simulink model "RM3_DD_PTO"  (R2019b)
settings: Solver=ode4  StartTime=0  StopTime=400  FixedStep=0.001  MaxStep=0.001  RelTol=1e-3  EnableMultiTasking=on
values from neighbouring files (symbols this model uses):
  ptosim = ptoSimClass('Direct Drive Linear Generator')    [ptoSimInputFile.m]
undefined symbols (not defined in the file or in its folder): body, constraint, pto
libraries: WECSim_Lib x5
settings Model: Creator=mlawson  LastModifiedBy=ahm_e
settings SolverCC: ZeroCrossControl=DisableAll  AlgebraicLoopSolver=LineSearch  AutoInsertRateTranBlk=on
settings DataIOCC: SaveFormat=Array  SaveOutput=off  SaveTime=off  ReturnWorkspaceOutputs=off
settings OptimizationCC: LifeSpan=inf
settings DebuggingCC: UnderspecifiedInitializationDetection=Classic  MergeDetectMultiDrivingBlocksExec=none  SolverPrmCheckMsg=warning  AllowSymbolicDim=off  StateNameClashWarn=warning  SFUnexpectedBacktrackingDiag=warning  SFNoUnconditionalDefaultTransitionDiag=warning  ArithmeticOperatorsInVariantConditions=warning
settings HardwareCC: ProdBitPerPointer=32  ProdBitPerSizeT=32  ProdBitPerPtrDiffT=32  ProdLargestAtomicFloat=None  ProdIntDivRoundTo=Undefined  ProdEndianess=Unspecified  ProdWordSize=32  ProdHWDeviceType=32-bit Generic
settings ModelReferenceCC: PropagateSignalLabelsOutOfModel=off
settings SFSimCC: SimUseLocalCustomCode=off  CustomCodeUndefinedFunction=UseInterfaceOnly
settings RTWCC: RTWUseLocalCustomCode=off
settings CodeAppCC: StateflowObjectComments=on
settings GRTTargetCC: TargetLangStandard=C89/C90 (ANSI)
settings ConfigComp: CovMetricSettings=dw  CovSaveCumulativeToWorkspaceVar=on  CovSaveSingleToWorkspaceVar=on  CovExternalEMLEnable=off  CovSFcnEnable=off
settings SimscapeCC: SimscapeNormalizeSystem=off
settings ConfigurationSet: Description=SimMechanics 2G
settings ExplorerConfigSet: InternalSimMechanicsExplorerSettings="<ExplorerConfiguration><canonicalview>default</canonicalview><TilePanel><TileInfo><Tiles Columns=\"1\" Count=\"1\" Rows=\"1\"><Column Left=\"2\" Weight=\"1\"/><Column Left=\"1335\"/><Row Top=\"2\" Weight=\"1\"/><Row Top=\"911\"/><Tile Height=\"1\" Width=\"1\" X=\"0\" Y=\"0\"/></Tiles></TileInfo><SceneInfo><SceneViewer><BGColor><R>0.60000002384185791</R><G>0.60000002384185791</G><B>0.60000002384185791</B></BGColor><Camera><Position><X>365.37645888990272</X><Y>-369.82486814446582</Y><Z>359.64809521743916</Z></Position><Center><X>-6.7351450971904585</X><Y>2.2867358426280204</Y><Z>-12.463508769654169</Z></Center><Up><X>-0.40824829046386307</X><Y>0.40824829046386307</Y><Z>0.81649658092772615</Z></Up><Left>-57.820127362122818</Left><Right>57.820127362122818</Right><Bottom>-38.308817187253304</Bottom><Top>38.308817187253304</Top></Camera></SceneViewer></SceneInfo></TilePanel></ExplorerConfiguration>"

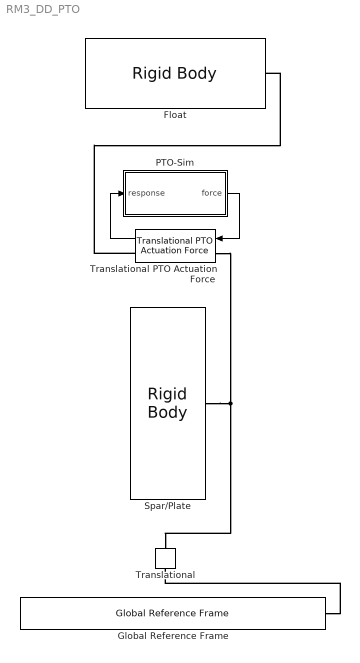
== system RM3_DD_PTO ==
  Float : WECSim_Lib/Body Elements/Rigid Body  body=body(1)
      settings: AttributesFormatString=%<body>  SourceProductName=WEC-Sim
  Global Reference Frame : WECSim_Lib/Frames/Global Reference Frame  waves=waves  simu=simu
      settings: SourceProductName=WEC-Sim
  PTO-Sim : Subsystem
  Spar/Plate : WECSim_Lib/Body Elements/Rigid Body  body=body(2)
      settings: AttributesFormatString=%<body>  SourceProductName=WEC-Sim
  Translational : WECSim_Lib/Constraints/Translational  constraint=constraint(1)
      settings: AttributesFormatString=%<constraint>  SourceProductName=WEC-Sim
  Translational PTO Actuation Force : WECSim_Lib/PTOs/Translational PTO Actuation Force  pto=pto(1)
      settings: AttributesFormatString=%<pto>  SourceProductName=WEC-Sim
  wires:
  Translational PTO Actuation Force/1 -> PTO-Sim/1(response)
  PTO-Sim/1(force) -> Translational PTO Actuation Force/1
  connections:
  Global Reference Frame/RConn1 -- Translational/LConn1
  Spar/Plate/RConn1 -- Translational PTO Actuation Force/LConn1 -- Translational/RConn1
  Translational PTO Actuation Force/RConn1 -- Float/RConn1

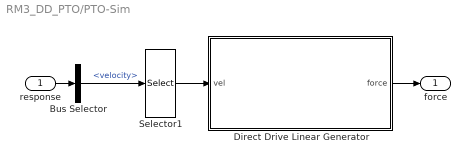
== system RM3_DD_PTO/PTO-Sim ==
  response : Inport
  Bus Selector : BusSelector  OutputSignals=velocity
  Direct Drive Linear Generator : Subsystem  AncestorBlock=PTOSim_Lib/Generator/Direct Drive Linear Generator  mask{ptosim=ptosim.pmLinearGenerator(1)}
      mask prompts: ptosim "Machine Name:"
      mask init:
      | if exist ('ptosim','var')
      |     h = [gcb '/To Workspace'];
      |     responseName = ['pmLinearGenerator' num2str(ptosim.number) '_out'];
      |     set_param(h,'VariableName',responseName);
      |     if ischar(ptosim.Rs)==1 ...
      |        || ischar(ptosim.Bfric)==1 ...
      |        || ischar(ptosim.tau_p)==1 ...
      |        || ischar(ptosim.lambda_fd)==1 ...
      |        || ischar(ptosim.Ls)==1 ...
      |        || ischar(ptosim.theta_d_0)==1 ...
      |        || ischar(ptosim.lambda_sq_0)==1 ...
      |        || ischar(ptosim.lambda_sd_0)==1 ...
      |        || ischar(ptosim.Rload) ==1
      |           error('One of the linear generator variables is undefined. For example, ptosim.pmLinearGenerator.variableName')
      |     end       
      | end
      | clear h responseName
  Selector1 : Selector  InputPortWidth=6  IndexOptions=Index vector (dialog)  Indices=3  OutputSizes=1
  force : Outport  VectorParamsAs1DForOutWhenUnconnected=off
  wires:
  Direct Drive Linear Generator/1(force) -> force/1
  response/1 -> Bus Selector/1
  Bus Selector/1 -> Selector1/1  "<velocity>"
  Selector1/1 -> Direct Drive Linear Generator/1(vel)

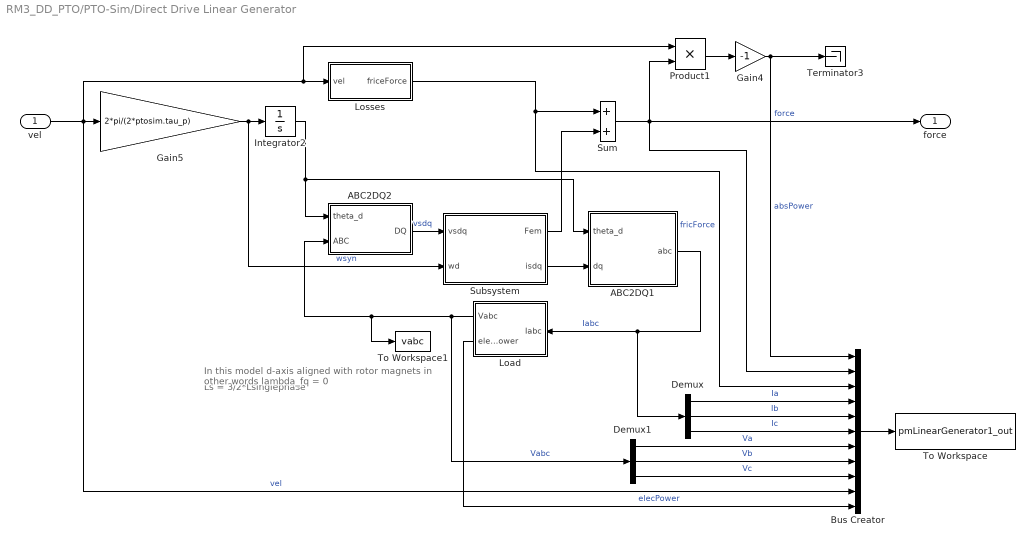
== system RM3_DD_PTO/PTO-Sim/Direct Drive Linear Generator ==
  note: Ls = 3/2*Lsinglephase
  note: In this model d-axis aligned with rotor magnets
      | in other words lambda_fq = 0
  vel : Inport
  ABC2DQ1 : Subsystem
  ABC2DQ2 : Subsystem
  Bus Creator : BusCreator  Inputs=11
  Demux : Demux  Outputs=3
  Demux1 : Demux  Outputs=3
  Gain4 : Gain  Gain=-1
  Gain5 : Gain  Gain=2*pi/(2*ptosim.tau_p)
  Integrator2 : Integrator  InitialCondition=ptosim.theta_d_0
  Load : Subsystem
  Losses : Subsystem
  Product1 : Product
  Subsystem : Subsystem
  Sum : Sum
  Terminator3 : Terminator
  To Workspace : ToWorkspace  VariableName=pmLinearGenerator1_out  SaveFormat=Structure With Time  SampleTime=-1
      settings: Decimation=round(simu.dtOut/simu.dt,0)
  To Workspace1 : ToWorkspace  VariableName=vabc  SaveFormat=Timeseries  SampleTime=-1
  force : Outport
  wires:
  Load/2(elecPower) -> Bus Creator/11  "elecPower"
  Demux1/3 -> Bus Creator/9  "Vc"
  Demux1/2 -> Bus Creator/8  "Vb"
  Demux1/1 -> Bus Creator/7  "Va"
  Demux/3 -> Bus Creator/6  "Ic"
  Demux/2 -> Bus Creator/5  "Ib"
  Demux/1 -> Bus Creator/4  "Ia"
  Bus Creator/1 -> To Workspace/1
  vel/1 -> Gain5/1, Product1/1, Losses/1(vel), Bus Creator/10  "vel"
  Load/1(Vabc) -> To Workspace1/1, ABC2DQ2/2(ABC), Demux1/1  "Vabc"
  Sum/1 -> force/1, Product1/2, Bus Creator/2  "force"
  Losses/1(friceForce) -> Sum/1, Bus Creator/3  "fricForce"
  Subsystem/2(isdq) -> ABC2DQ1/2(dq)
  Subsystem/1(Fem) -> Sum/2
  Gain4/1 -> Terminator3/1, Bus Creator/1  "absPower"
  Product1/1 -> Gain4/1
  Integrator2/1 -> ABC2DQ1/1(theta_d), ABC2DQ2/1(theta_d)
  Gain5/1 -> Integrator2/1, Subsystem/2(wd)  "wsyn"
  ABC2DQ1/1(abc) -> Load/1(Iabc), Demux/1  "Iabc"
  ABC2DQ2/1(DQ) -> Subsystem/1(vsdq)  "vsdq"

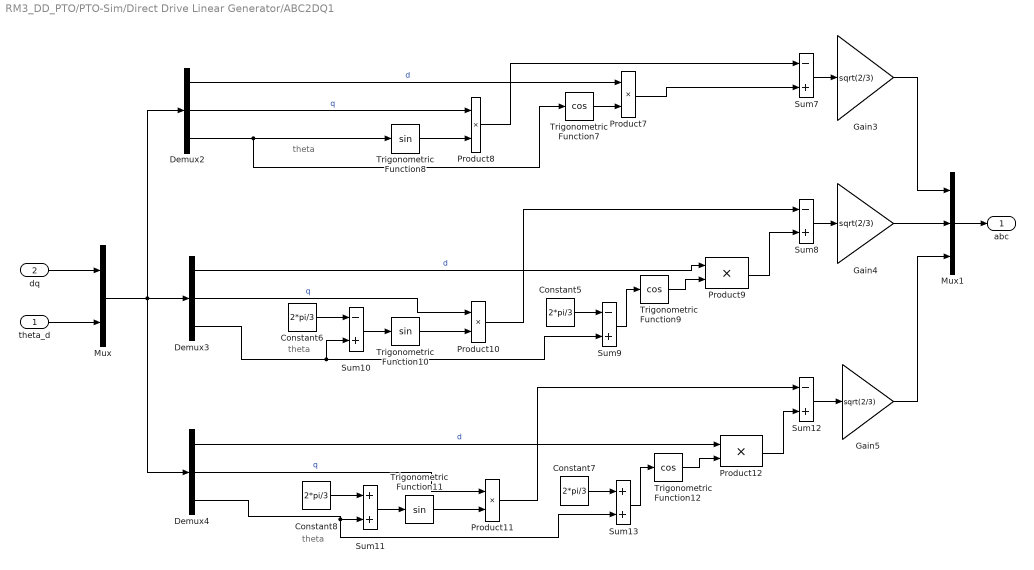
== system RM3_DD_PTO/PTO-Sim/Direct Drive Linear Generator/ABC2DQ1 ==
  note: theta
  note: theta
  note: theta
  theta_d : Inport
  dq : Inport  Port=2
  Constant{5..8} (4 alike) : Constant  Value=2*pi/3
  Demux2 : Demux  Outputs=3
      settings: DisplayOption=none
  Demux3 : Demux  Outputs=3
      settings: DisplayOption=none
  Demux4 : Demux  Outputs=3
      settings: DisplayOption=none
  Gain3 : Gain  Gain=sqrt(2/3)  SaturateOnIntegerOverflow=on  OutDataTypeStr=Inherit: Same as input  ParamDataTypeStr=Inherit: Same as input
  Gain4 : Gain  Gain=sqrt(2/3)  SaturateOnIntegerOverflow=on  OutDataTypeStr=Inherit: Same as input  ParamDataTypeStr=Inherit: Same as input
  Gain5 : Gain  Gain=sqrt(2/3)  SaturateOnIntegerOverflow=on  OutDataTypeStr=Inherit: Same as input  ParamDataTypeStr=Inherit: Same as input
  Mux : Mux  Inputs=2
  Mux1 : Mux  Inputs=3
  Product{7..12} (6 alike) : Product  InputSameDT=on  SaturateOnIntegerOverflow=on  OutDataTypeStr=Inherit: Same as first input
  Sum{7..10,12} (5 alike) : Sum  Inputs=-+  InputSameDT=on  SaturateOnIntegerOverflow=on  OutDataTypeStr=Inherit: Same as first input
  Sum11 : Sum  InputSameDT=on  SaturateOnIntegerOverflow=on  OutDataTypeStr=Inherit: Same as first input
  Sum13 : Sum  InputSameDT=on  SaturateOnIntegerOverflow=on  OutDataTypeStr=Inherit: Same as first input
  Trigonometric Function10 : Trigonometry
  Trigonometric Function11 : Trigonometry
  Trigonometric Function12 : Trigonometry  Operator=cos
  Trigonometric Function7 : Trigonometry  Operator=cos
  Trigonometric Function8 : Trigonometry
  Trigonometric Function9 : Trigonometry  Operator=cos
  abc : Outport
  wires:
  Trigonometric Function8/1 -> Product8/2
  Gain5/1 -> Mux1/3
  Gain4/1 -> Mux1/2
  Gain3/1 -> Mux1/1
  Sum12/1 -> Gain5/1
  Sum8/1 -> Gain4/1
  Sum7/1 -> Gain3/1
  Constant8/1 -> Sum11/1
  Sum11/1 -> Trigonometric Function11/1
  Constant7/1 -> Sum13/1
  Sum13/1 -> Trigonometric Function12/1
  Demux4/2 -> Product11/1  "q"
  Trigonometric Function11/1 -> Product11/2
  Demux4/3 -> Sum11/2, Sum13/2
  Product11/1 -> Sum12/1
  Product12/1 -> Sum12/2
  Demux4/1 -> Product12/1  "d"
  Trigonometric Function12/1 -> Product12/2
  Constant6/1 -> Sum10/1
  Sum10/1 -> Trigonometric Function10/1
  Constant5/1 -> Sum9/1
  Sum9/1 -> Trigonometric Function9/1
  Demux3/2 -> Product10/1  "q"
  Trigonometric Function10/1 -> Product10/2
  Demux3/3 -> Sum9/2, Sum10/2
  Product10/1 -> Sum8/1
  Product9/1 -> Sum8/2
  Demux3/1 -> Product9/1  "d"
  Trigonometric Function9/1 -> Product9/2
  Demux2/2 -> Product8/1  "q"
  Demux2/3 -> Trigonometric Function7/1, Trigonometric Function8/1
  Product8/1 -> Sum7/1
  Product7/1 -> Sum7/2
  Demux2/1 -> Product7/1  "d"
  Trigonometric Function7/1 -> Product7/2
  Mux/1 -> Demux3/1, Demux2/1, Demux4/1
  theta_d/1 -> Mux/2
  dq/1 -> Mux/1
  Mux1/1 -> abc/1

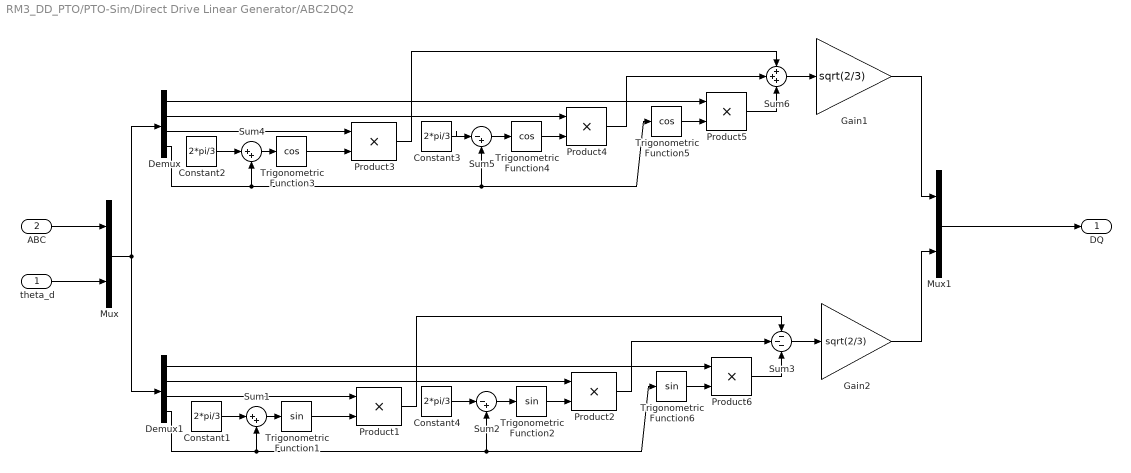
== system RM3_DD_PTO/PTO-Sim/Direct Drive Linear Generator/ABC2DQ2 ==
  theta_d : Inport
  ABC : Inport  Port=2
  Constant{1..4} (4 alike) : Constant  Value=2*pi/3
  Demux : Demux
      settings: DisplayOption=none
  Demux1 : Demux
      settings: DisplayOption=none
  Gain1 : Gain  Gain=sqrt(2/3)  SaturateOnIntegerOverflow=on  OutDataTypeStr=Inherit: Same as input  ParamDataTypeStr=Inherit: Same as input
  Gain2 : Gain  Gain=sqrt(2/3)  SaturateOnIntegerOverflow=on  OutDataTypeStr=Inherit: Same as input  ParamDataTypeStr=Inherit: Same as input
  Mux : Mux  Inputs=2
  Mux1 : Mux  Inputs=2
  Product{1..6} (6 alike) : Product  InputSameDT=on  SaturateOnIntegerOverflow=on  OutDataTypeStr=Inherit: Same as first input
  Sum1 : Sum  Inputs=|++  InputSameDT=on  SaturateOnIntegerOverflow=on  OutDataTypeStr=Inherit: Same as first input
  Sum2 : Sum  Inputs=|-+  InputSameDT=on  SaturateOnIntegerOverflow=on  OutDataTypeStr=Inherit: Same as first input
  Sum3 : Sum  Inputs=---  InputSameDT=on  SaturateOnIntegerOverflow=on  OutDataTypeStr=Inherit: Same as first input
  Sum4 : Sum  Inputs=|++  InputSameDT=on  SaturateOnIntegerOverflow=on  OutDataTypeStr=Inherit: Same as first input
  Sum5 : Sum  Inputs=|-+  InputSameDT=on  SaturateOnIntegerOverflow=on  OutDataTypeStr=Inherit: Same as first input
  Sum6 : Sum  Inputs=+++  InputSameDT=on  SaturateOnIntegerOverflow=on  OutDataTypeStr=Inherit: Same as first input
  Trigonometric Function1 : Trigonometry
  Trigonometric Function2 : Trigonometry
  Trigonometric Function3 : Trigonometry  Operator=cos
  Trigonometric Function4 : Trigonometry  Operator=cos
  Trigonometric Function5 : Trigonometry  Operator=cos
  Trigonometric Function6 : Trigonometry
  DQ : Outport
  wires:
  Sum1/1 -> Trigonometric Function1/1
  Demux1/4 -> Sum2/2, Trigonometric Function6/1, Sum1/2
  Demux1/3 -> Product1/1
  Demux1/2 -> Product2/1
  Demux1/1 -> Product6/1
  Gain2/1 -> Mux1/2
  Trigonometric Function1/1 -> Product1/2
  Product2/1 -> Sum3/2
  Product1/1 -> Sum3/1
  Sum3/1 -> Gain2/1
  Constant4/1 -> Sum2/1
  Trigonometric Function6/1 -> Product6/2
  Trigonometric Function2/1 -> Product2/2
  Sum2/1 -> Trigonometric Function2/1
  Constant1/1 -> Sum1/1
  Product6/1 -> Sum3/3
  Sum4/1 -> Trigonometric Function3/1
  Mux/1 -> Demux1/1, Demux/1
  Demux/4 -> Sum4/2, Trigonometric Function5/1, Sum5/2
  Demux/3 -> Product3/1
  Demux/2 -> Product4/1
  Demux/1 -> Product5/1
  theta_d/1 -> Mux/2
  ABC/1 -> Mux/1
  Gain1/1 -> Mux1/1
  Trigonometric Function3/1 -> Product3/2
  Product4/1 -> Sum6/2
  Product3/1 -> Sum6/1
  Sum6/1 -> Gain1/1
  Constant3/1 -> Sum5/1
  Trigonometric Function5/1 -> Product5/2
  Trigonometric Function4/1 -> Product4/2
  Sum5/1 -> Trigonometric Function4/1
  Constant2/1 -> Sum4/1
  Product5/1 -> Sum6/3
  Mux1/1 -> DQ/1

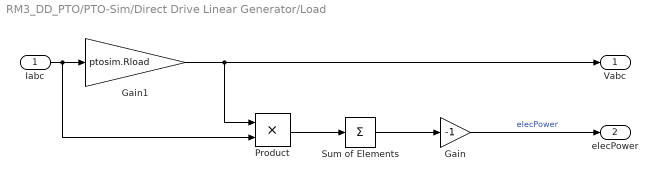
== system RM3_DD_PTO/PTO-Sim/Direct Drive Linear Generator/Load ==
  Iabc : Inport
  Gain : Gain  Gain=-1
  Gain1 : Gain  Gain=ptosim.Rload
  Product : Product
  Sum of Elements : Sum  Inputs=+
  Vabc : Outport
  elecPower : Outport  Port=2
  wires:
  Sum of Elements/1 -> Gain/1
  Iabc/1 -> Product/2, Gain1/1
  Product/1 -> Sum of Elements/1
  Gain1/1 -> Vabc/1, Product/1
  Gain/1 -> elecPower/1  "elecPower"

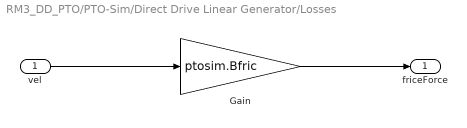
== system RM3_DD_PTO/PTO-Sim/Direct Drive Linear Generator/Losses ==
  vel : Inport
  Gain : Gain  Gain=ptosim.Bfric
  friceForce : Outport
  wires:
  Gain/1 -> friceForce/1
  vel/1 -> Gain/1

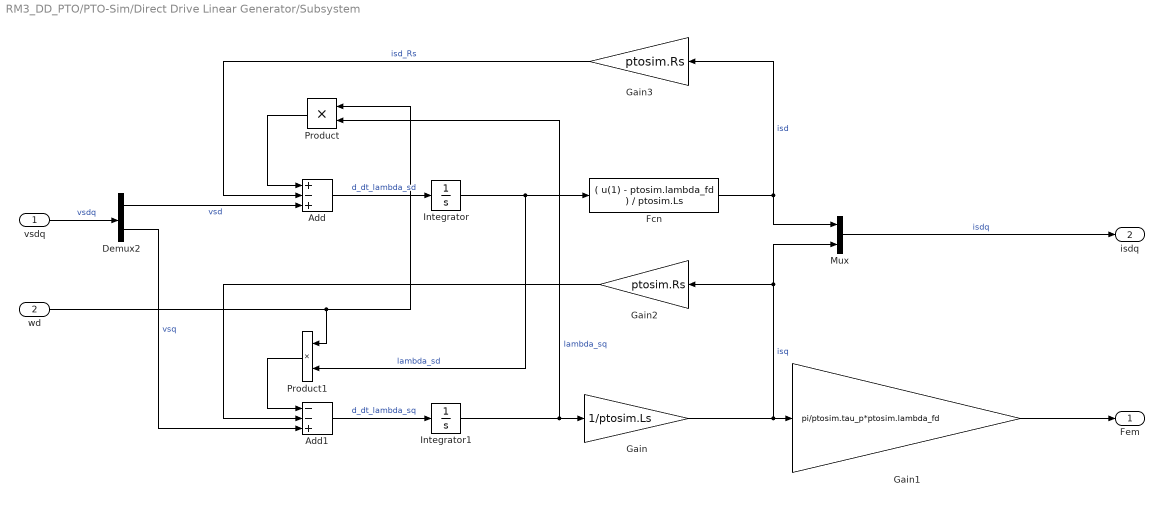
== system RM3_DD_PTO/PTO-Sim/Direct Drive Linear Generator/Subsystem ==
  vsdq : Inport
  wd : Inport  Port=2
  Add : Sum  Inputs=+-+
  Add1 : Sum  Inputs=--+
  Demux2 : Demux  Outputs=2
      settings: DisplayOption=none
  Fcn : Fcn  Expr=( u(1) - ptosim.lambda_fd ) / ptosim.Ls
  Gain : Gain  Gain=1/ptosim.Ls
  Gain1 : Gain  Gain=pi/ptosim.tau_p*ptosim.lambda_fd
  Gain2 : Gain  Gain=ptosim.Rs
  Gain3 : Gain  Gain=ptosim.Rs
  Integrator : Integrator  InitialCondition=ptosim.lambda_sd_0
  Integrator1 : Integrator  InitialCondition=ptosim.lambda_sq_0
  Mux : Mux  Inputs=2
  Product : Product  RndMeth=Zero
  Product1 : Product  RndMeth=Zero
  Fem : Outport
  isdq : Outport  Port=2
  wires:
  Gain1/1 -> Fem/1
  Mux/1 -> isdq/1  "isdq"
  Gain2/1 -> Add1/2
  Gain3/1 -> Add/2  "isd_Rs"
  vsdq/1 -> Demux2/1  "vsdq"
  Demux2/2 -> Add1/3  "vsq"
  Demux2/1 -> Add/3  "vsd"
  Product1/1 -> Add1/1
  Gain/1 -> Gain1/1, Mux/2, Gain2/1  "isq"
  wd/1 -> Product/1, Product1/1
  Integrator1/1 -> Product/2, Gain/1  "lambda_sq"
  Add1/1 -> Integrator1/1  "d_dt_lambda_sq"
  Product/1 -> Add/1
  Fcn/1 -> Mux/1, Gain3/1  "isd"
  Integrator/1 -> Fcn/1, Product1/2  "lambda_sd"
  Add/1 -> Integrator/1  "d_dt_lambda_sd"
